simulink model "inverted_pendulum_simulink"  (R2025a)
settings: Solver=VariableStepAuto  StartTime=0.0  StopTime=10  MaxStep=1e-3  RelTol=1e-3
values from neighbouring files (symbols this model uses):
  g = 9.81    [inverted_pendulum.m]
  l = 0.36    [inverted_pendulum.m]
  M = 2.4    [inverted_pendulum.m]
  m = 0.23    [inverted_pendulum.m]
  theta_0 = 0.05    [inverted_pendulum.m]
settings Model: Creator=Emre  LastModifiedBy=Emre

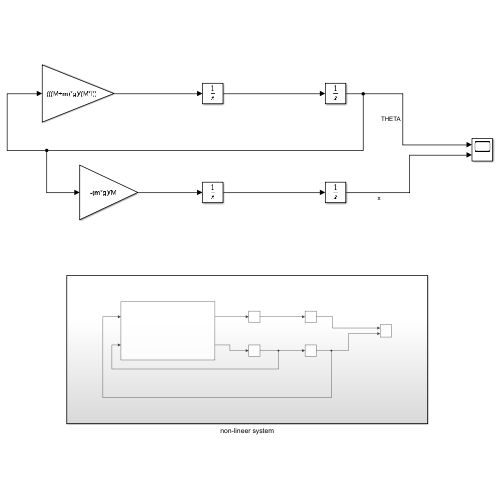
[thumbnail: Simulink's stored preview of the top-level diagram]
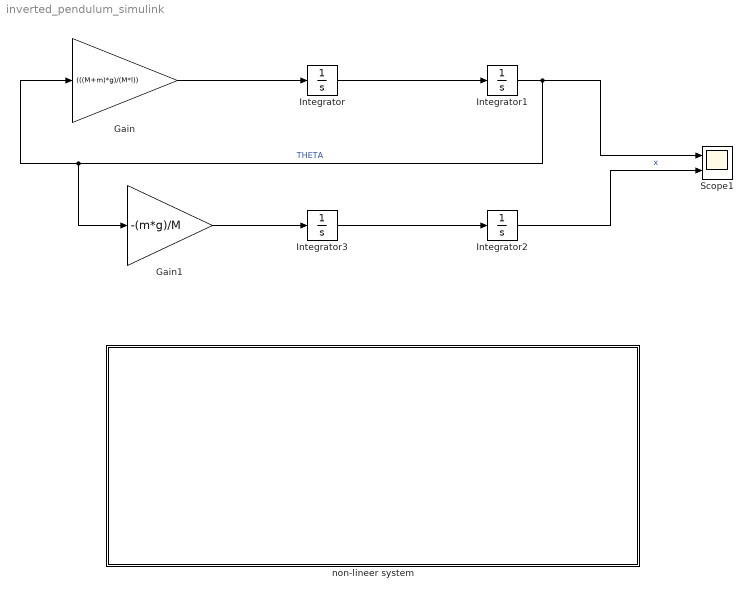
== system inverted_pendulum_simulink ==
  Gain : Gain  Gain=(((M+m)*g)/(M*l))
  Gain1 : Gain  Gain=-(m*g)/M
  Integrator : Integrator
  Integrator1 : Integrator  InitialCondition=theta_0
  Integrator2 : Integrator
  Integrator3 : Integrator
  Scope1 : Scope  NumInputPorts=2
      settings: ActiveDisplayYMinimum=-2.165175731082242E+21  ActiveDisplayYMaximum=1.5237315153250264E+22
  non-lineer system : Subsystem
  wires:
  Integrator1/1 -> Gain/1, Gain1/1, Scope1/1  "THETA"
  Integrator2/1 -> Scope1/2  "x"
  Integrator3/1 -> Integrator2/1
  Gain1/1 -> Integrator3/1
  Integrator/1 -> Integrator1/1
  Gain/1 -> Integrator/1

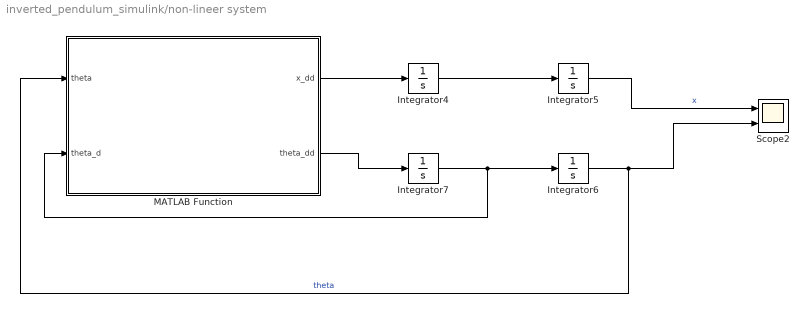
== system inverted_pendulum_simulink/non-lineer system ==
  Integrator4 : Integrator
  Integrator5 : Integrator
  Integrator6 : Integrator  InitialCondition=theta_0
  Integrator7 : Integrator
  MATLAB Function : MATLAB Function  TreatAsAtomicUnit=on
  Scope2 : Scope  NumInputPorts=2
      settings: ActiveDisplayYMinimum=-0.81279622874136037  ActiveDisplayYMaximum=7.0160721431790778  DataLoggingVariableName=ScopeData2
  wires:
  MATLAB Function/1(x_dd) -> Integrator4/1
  Integrator6/1 -> Scope2/2, MATLAB Function/1(theta)  "theta"
  Integrator7/1 -> MATLAB Function/2(theta_d), Integrator6/1
  Integrator4/1 -> Integrator5/1
  Integrator5/1 -> Scope2/1  "x"
  MATLAB Function/2(theta_dd) -> Integrator7/1

== matlab function inverted_pendulum_simulink/non-lineer system/MATLAB Function ==
  data: theta input; x_dd output; theta_d input; theta_dd output
function [x_dd, theta_dd] = non_lineer_model(theta, theta_d)
    % Parametreler (Workspace'ten de çekilebilir ama buraya yazmak en risksizidir)
    M = 2.4; 
    m = 0.23;
    l = 0.36;
    g = 9.81;

    % Ortak payda (Formül kalabalığını azaltmak için)
    payda = M + m * (sin(theta))^2;

    % İvme Denklemleri
    x_dd = (m * sin(theta) * (l * theta_d^2 - g * cos(theta))) / payda;
    theta_dd = ((M + m) * g * sin(theta) - m * l * theta_d^2 * sin(theta) * cos(theta)) / (l * payda);
end
